simulink model "pid_ciagly"  (R2022a)
settings: Solver=VariableStepAuto  StartTime=0.0  StopTime=100  RelTol=1e-3
values from neighbouring files (symbols this model uses):
  Kp = 0.408    [dane.m]
  Td = 1.859    [PID_dysrk.m]    (also in dane.m = 1.1859)
  Ti = 7.748    [PID_dysrk.m]    (also in dane.m)
settings Model: Creator=danie  LastModifiedBy=danie

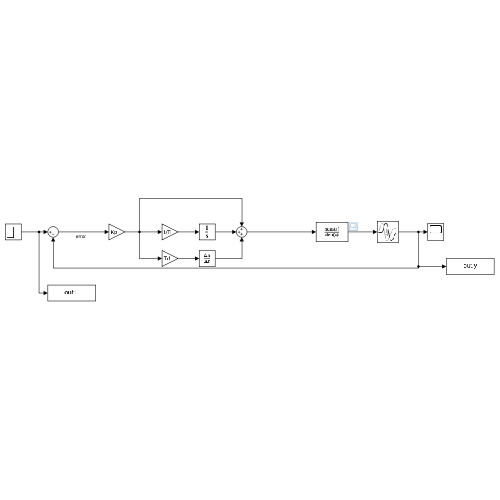
[thumbnail: Simulink's stored preview of the top-level diagram]
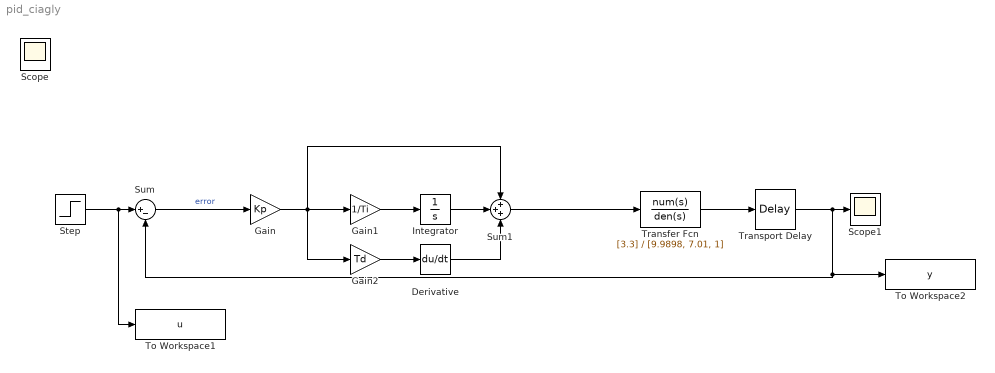
== system pid_ciagly ==
  Derivative : Derivative
  Gain : Gain  Gain=Kp
  Gain1 : Gain  Gain=1/Ti
  Gain2 : Gain  Gain=Td
  Integrator : Integrator
  Scope1 : Scope
  Step : Step  SampleTime=0
  Sum : Sum  Inputs=|+-
  Sum1 : Sum  Inputs=+++
  To Workspace1 : ToWorkspace  VariableName=u  SaveFormat=Timeseries  SampleTime=-1
  To Workspace2 : ToWorkspace  VariableName=y  SaveFormat=Timeseries  SampleTime=-1
  Transfer Fcn : TransferFcn  Numerator=[3.3]  Denominator=[9.9898, 7.01, 1]
  Transport Delay : TransportDelay  DelayTime=5
  Scope : Scope
  wires:
  Step/1 -> To Workspace1/1, Sum/1
  Sum1/1 -> Transfer Fcn/1
  Transfer Fcn/1 -> Transport Delay/1
  Transport Delay/1 -> To Workspace2/1, Sum/2, Scope1/1
  Gain/1 -> Gain1/1, Sum1/1, Gain2/1
  Derivative/1 -> Sum1/3
  Integrator/1 -> Sum1/2
  Sum/1 -> Gain/1  "error"
  Gain2/1 -> Derivative/1
  Gain1/1 -> Integrator/1
